simulink model "dc_ac_inverter_sim"  (R2021a)
settings: Solver=VariableStepAuto  StartTime=0.0  StopTime=10.0  RelTol=1e-3
libraries: simulink x1
settings Model: Creator=st241021  LastModifiedBy=st241021

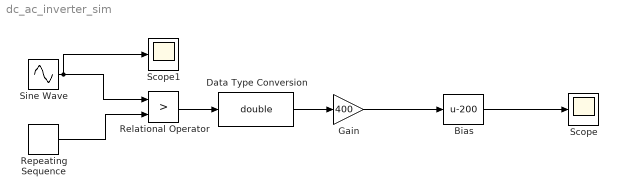
== system dc_ac_inverter_sim ==
  Bias : Bias  Bias=-200
  Data Type Conversion : DataTypeConversion  OutDataTypeStr=double
  Gain : Gain  Gain=400
  Relational Operator : RelationalOperator  Operator=>  OutDataTypeStr=boolean  RndMeth=Simplest
  Repeating Sequence : simulink/Sources/Repeating Sequence  rep_seq_t=[0 0.01]  rep_seq_y=[-1 1]
  Scope : Scope
  Scope1 : Scope
  Sine Wave : Sin  Frequency=2*pi*50  SampleTime=0
  wires:
  Sine Wave/1 -> Scope1/1, Relational Operator/1
  Repeating Sequence/1 -> Relational Operator/2
  Gain/1 -> Bias/1
  Bias/1 -> Scope/1
  Relational Operator/1 -> Data Type Conversion/1
  Data Type Conversion/1 -> Gain/1
